simulink model "Properties_Controller_Tank_2_Primitives"  (R2012b)
settings: Solver=FixedStepDiscrete  StartTime=0.0  StopTime=10.0  FixedStep=0.1  RelTol=1e-3
settings Model: Creator=Kerianne  LastModifiedBy=Kerianne
settings DataIOCC: SaveFormat=Structure
settings OptimizationCC: InlineParams=on

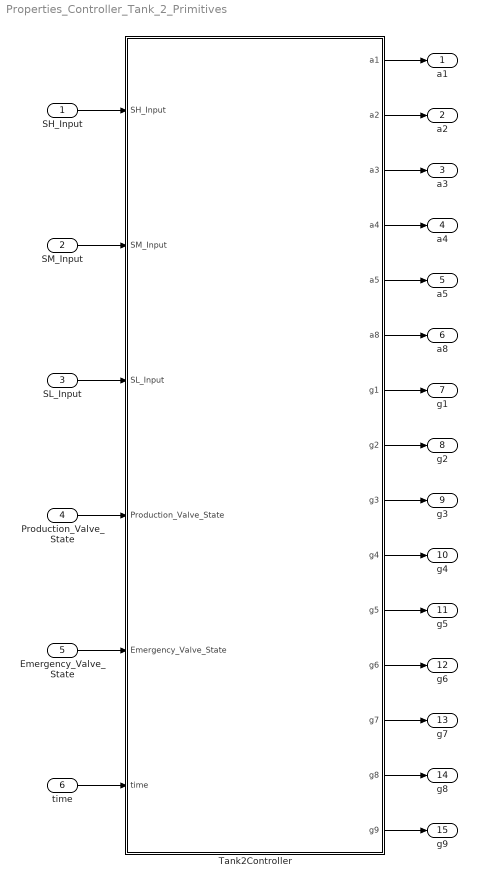
== system Properties_Controller_Tank_2_Primitives ==
  SH_Input : Inport
  SM_Input : Inport  Port=2
  SL_Input : Inport  Port=3
  Production_Valve_State : Inport  Port=4
  Emergency_Valve_State : Inport  Port=5
  time : Inport  Port=6
  Tank2Controller : MATLAB Function  TreatAsAtomicUnit=on
  a1 : Outport
  a2 : Outport  Port=2
  a3 : Outport  Port=3
  a4 : Outport  Port=4
  a5 : Outport  Port=5
  a8 : Outport  Port=6
  g1 : Outport  Port=7
  g2 : Outport  Port=8
  g3 : Outport  Port=9
  g4 : Outport  Port=10
  g5 : Outport  Port=11
  g6 : Outport  Port=12
  g7 : Outport  Port=13
  g8 : Outport  Port=14
  g9 : Outport  Port=15
  wires:
  Production_Valve_State/1 -> Tank2Controller/4(Production_Valve_State)
  Emergency_Valve_State/1 -> Tank2Controller/5(Emergency_Valve_State)
  SH_Input/1 -> Tank2Controller/1(SH_Input)
  time/1 -> Tank2Controller/6(time)
  SM_Input/1 -> Tank2Controller/2(SM_Input)
  SL_Input/1 -> Tank2Controller/3(SL_Input)
  Tank2Controller/1(a1) -> a1/1
  Tank2Controller/14(g8) -> g8/1
  Tank2Controller/5(a5) -> a5/1
  Tank2Controller/4(a4) -> a4/1
  Tank2Controller/3(a3) -> a3/1
  Tank2Controller/2(a2) -> a2/1
  Tank2Controller/13(g7) -> g7/1
  Tank2Controller/12(g6) -> g6/1
  Tank2Controller/11(g5) -> g5/1
  Tank2Controller/10(g4) -> g4/1
  Tank2Controller/9(g3) -> g3/1
  Tank2Controller/8(g2) -> g2/1
  Tank2Controller/7(g1) -> g1/1
  Tank2Controller/15(g9) -> g9/1
  Tank2Controller/6(a8) -> a8/1

== matlab function Properties_Controller_Tank_2_Primitives/Tank2Controller ==
  data: SH_Input input; a1 output; SM_Input input; SL_Input input; Production_Valve_State input; Emergency_Valve_State input; a2 output; a3 output; a4 output; a5 output; a8 output; g1 output; g2 output; g3 output; g4 output; g5 output; g6 output; g7 output; g8 output; time input; g9 output
function [a1, a2, a3, a4, a5, a8, g1, g2, g3, g4, g5, g6, g7, g8, g9] = verification_condition(SH_Input, SM_Input, SL_Input, Production_Valve_State, Emergency_Valve_State, time)
% Tank 2 Controller Design Verifier
% Last Updated 23 Feb 2015
% Based on 2015 02 06 Controller.aadl

%% Persistent Variables
persistent Pre_E_Valve_State
if isempty(Pre_E_Valve_State)
    Pre_E_Valve_State = 0;
end
Pre_E_Valve_State = Emergency_Valve_State;
persistent Pre_P_Valve_State
if isempty(Pre_P_Valve_State)
    Pre_P_Valve_State = 0;
end
Pre_P_Valve_State = Production_Valve_State;
%% Assumptions
% assume "If the high sensor is true, then the mid sensor is True" :		
a1 = implies(SH_Input, SM_Input);
% assume "If the mid sensor is true, then the low sensor is True"
a2 = implies(SM_Input, SL_Input);
% assume "SH_Input is 0 (false) or 1(true)"
a3 = sensor_0_or_1(SH_Input);
% assume "SM_Input is 0 (false) or 1(true)"
a4 = sensor_0_or_1(SM_Input);
% assume "SL_Input is 0 (false) or 1(true)"
a5 = sensor_0_or_1(SL_Input);
% assume "The Prev_P_Valve is the same as the output Valve_Output_P_State 
% % in the previous step" 
% a6 = prev_P_Valve_State == Pre_P_Valve_State;
% % assume "The Prev_E_Valve is the same as the output Valve_Output_E_State 
% % in the previous step" 
% a7 = prev_E_Valve_State == Pre_E_Valve_State;
% assume "The sensors are all initially false (The tanks are initially
% empty)
a8 = init_sensors_false(SM_Input,SH_Input,SL_Input,time);

%% Guarantees
% guarantee "The output emergency valve is initially closed"  
g1 = e_valve_initially_closed(Emergency_Valve_State, time);
% guarantee "The output production valve is initially closed"
g2 = p_valve_initially_closed(Production_Valve_State, time);
% guarantee "When SL_Input is False, the valves shall be Closed" : 
g3 = sl_input_false_cond(SL_Input, Production_Valve_State, Emergency_Valve_State);
% guarantee "When SM_Input is False and the SL_Input is true, the production valve shall be open and the emergency valve shall be closed" : 
g4 = sl_true_sm_false_cond(SL_Input, SM_Input, Production_Valve_State, Emergency_Valve_State);
% guarantee "When the SH_Input is true, both valves will be open" 
g5 = sh_input_true_cond(SH_Input, Production_Valve_State, Emergency_Valve_State);
% guarantee "When the SM_Input is True and the SH_Input is False and the emergency valve was previously open, the valves shall be Open" 
g6 = sm_true_sh_false_preE_true_cond(SM_Input, SH_Input, Production_Valve_State, Emergency_Valve_State, Pre_E_Valve_State);			
% guarantee "When the SM_Input is True and the SH_Input is False and the emergency valve was previously closed, the production valve shall be open and the emergency valve shall be closed" : 
g7 = sm_true_sh_false_preE_false_cond(SM_Input, SH_Input, Production_Valve_State, Emergency_Valve_State, Pre_E_Valve_State);	
% guarantee "Production Valve State is 0 (closed) or 1 (open)"
g8 = actuator_0_or_1(Production_Valve_State);
% guarantee "Emergency Valve State is 0 (closed) or 1 (open)"
g9 = actuator_0_or_1(Emergency_Valve_State);

% a1 - a2
function c = implies(a,b)      
     c = ((not (a)) || b);
%for a3-a5
function result = sensor_0_or_1(sensor)
    result = (sensor == 0 | sensor == 1);
function result = init_sensors_false(SM_Input,SH_Input,SL_Input,time)
    UnderThisCondition = (time == 0);
    ResultShouldBe = (SM_Input == 0 && SH_Input == 0 && SL_Input == 0);
    result = implies(UnderThisCondition, ResultShouldBe);
%for g1
function result = e_valve_initially_closed(Emergency_Valve_State, time)
    UnderThisCondition = (time == 0);
    ResultShouldBe = (Emergency_Valve_State == 0);
    result = implies(UnderThisCondition, ResultShouldBe);
%for g2
function result = p_valve_initially_closed(Production_Valve_State, time)
    UnderThisCondition = (time == 0);
    ResultShouldBe = (Production_Valve_State == 0);
    result = implies(UnderThisCondition, ResultShouldBe);
%for g3 
function result = sl_input_false_cond(SL_Input, Production_Valve_State, Emergency_Valve_State) 
    UnderThisCondition = (SL_Input == 0);
    ResultShouldBe = (Production_Valve_State == 0) && (Emergency_Valve_State == 0);
    result = implies(UnderThisCondition, ResultShouldBe); 
%for g4
function result = sl_true_sm_false_cond(SL_Input, SM_Input, Production_Valve_State, Emergency_Valve_State) 
    UnderThisCondition = (SL_Input == 1) && (SM_Input == 0);
    ResultShouldBe = (Production_Valve_State == 1) && (Emergency_Valve_State == 0);
    result = implies(UnderThisCondition, ResultShouldBe); 
%for g5
function result = sh_input_true_cond(SH_Input, Production_Valve_State, Emergency_Valve_State) 
    UnderThisCondition = (SH_Input == 1);
    ResultShouldBe = (Production_Valve_State == 1) && (Emergency_Valve_State == 1);
    result = implies(UnderThisCondition, ResultShouldBe); 
%for g6
function result = sm_true_sh_false_preE_true_cond(SM_Input, SH_Input, Production_Valve_State, Emergency_Valve_State, Pre_E_Valve_State)
    UnderThisCondition = (SM_Input == 1) && (SH_Input == 0) && (Pre_E_Valve_State == 1);
    ResultShouldBe = (Production_Valve_State == 1) && (Emergency_Valve_State == 1);
    result = implies(UnderThisCondition, ResultShouldBe);   
%for g7
function result = sm_true_sh_false_preE_false_cond(SM_Input, SH_Input, Production_Valve_State, Emergency_Valve_State, Pre_E_Valve_State)
    UnderThisCondition = (SM_Input == 1) && (SH_Input == 0) && (Pre_E_Valve_State == 0);
    ResultShouldBe = (Production_Valve_State == 1) && (Emergency_Valve_State == 0);
    result = implies(UnderThisCondition, ResultShouldBe);		
%for g8 & g9			
function result = actuator_0_or_1(actuator)
    result = (actuator == 0 | actuator == 1);

% % assume "Production Valve State is 0 (closed) or 1 (open)"
% a6 = actuator_0_or_1(Production_Valve_State);
% % assume " Emergency Valve State is 0 (closed) or 1 (open)"
% a7 = actuator_0_or_1(Emergency_Valve_State);
% 
% % Additional Assumptions
% % assume "the tank is initally empty in form of all sensor false"
% a8 = sensors_initially_false(SH_Input,SM_Input, SL_Input, time);
% 
% % guarantee "When the SM_Input is True and the SH_Input is False and the emergency valve was previously open, and the input valve is open, then the valves shall be Open" : 
% g6 = sm_true_sh_false_preE_true_cond(SM_Input, SH_Input, Production_Valve_State, Emergency_Valve_State, Pre_E_Valve_State, Valve_Input_State);			
% 


% function c = implies(a,b)      
%      c = ((not (a)) || b);
% 
% %for a2-a5
% function result = sensor_0_or_1(sensor)
%     result = (sensor == 0 | sensor == 1);
% %for a6-a7

% function result = sensors_initially_false(SH_Input,SM_Input, SL_Input, time)
%     UnderThisCondition = (time == 0.0);
%     ResultShouldBe = (SH_Input == 0 && SM_Input == 0 && SL_Input == 0);
%     result = implies(UnderThisCondition, ResultShouldBe);   
%      
% %for g1
% function result = e_valve_initially_closed(Emergency_Valve_State, time)
%     UnderThisCondition = (time == 0);
%     ResultShouldBe = (Emergency_Valve_State == 0);
%     result = implies(UnderThisCondition, ResultShouldBe);
% %for g2
% function result = p_valve_initially_closed(Production_Valve_State, time)
%     UnderThisCondition = (time == 0);
%     ResultShouldBe = (Production_Valve_State == 0);
%     result = implies(UnderThisCondition, ResultShouldBe);
% %for g3 
% function result = sl_input_false_cond(SL_Input, Production_Valve_State, Emergency_Valve_State) 
%     UnderThisCondition = (SL_Input == 0);
%     ResultShouldBe = (Production_Valve_State == 0) && (Emergency_Valve_State == 0);
%     result = implies(UnderThisCondition, ResultShouldBe); 
% %for g4
% function result = sl_true_sm_false_cond(SL_Input, SM_Input, Production_Valve_State, Emergency_Valve_State) 
%     UnderThisCondition = (SL_Input == 1) && (SM_Input == 0);
%     ResultShouldBe = (Production_Valve_State == 1) && (Emergency_Valve_State == 0);
%     result = implies(UnderThisCondition, ResultShouldBe); 
% %for g5
% function result = sh_input_true_cond(SH_Input, Production_Valve_State, Emergency_Valve_State) 
%     UnderThisCondition = (SH_Input == 1);
%     ResultShouldBe = (Production_Valve_State == 1) && (Emergency_Valve_State == 1);
%     result = implies(UnderThisCondition, ResultShouldBe); 
% %for g6
% function result = sm_true_sh_false_preE_true_cond(SM_Input, SH_Input, Production_Valve_State, Emergency_Valve_State, Pre_E_Valve_State, Input_Valve_State)
%     UnderThisCondition = (SM_Input == 1) && (SH_Input == 0) && (Pre_E_Valve_State == 1) && (Input_Valve_State == 1);
%     ResultShouldBe = (Production_Valve_State == 1) && (Emergency_Valve_State == 1);
%     result = implies(UnderThisCondition, ResultShouldBe);   
% %for g7
% function result = sm_true_sh_false_preE_false_cond(SM_Input, SH_Input, Production_Valve_State, Emergency_Valve_State, Pre_E_Valve_State)
%     UnderThisCondition = (SM_Input == 1) && (SH_Input == 0) && (Pre_E_Valve_State == 0);
%     ResultShouldBe = (Production_Valve_State == 1) && (Emergency_Valve_State == 0);
%     result = implies(UnderThisCondition, ResultShouldBe);
